simulink model "Rear_SUS_S"  (R2014a)
settings: Solver=ode3  StartTime=0.0  StopTime=T  FixedStep=0.1  RelTol=1e-3
values from neighbouring files (symbols this model uses):
  CA = str2double(get(handles.CA,'string'))    [Rear_SUS.m]    (also in Rear_SUS_GUI.m)
  IN = str2double(get(handles.IN,'string'))    [Rear_SUS.m]    (also in Rear_SUS_GUI.m)
  LT = str2double(get(handles.LT,'string'))    [Rear_SUS_GUI.m]
  N = 1    [Rear_SUS.m]
  Rty = 0    [Rear_SUS_GUI.m]
  Rtz = 0    [Rear_SUS_GUI.m]
  SR = str2double(get(handles.SR,'string'))    [Rear_SUS.m]    (also in Rear_SUS_GUI.m)
  T5 = str2double(get(handles.T5,'string'))    [Rear_SUS.m]    (also in Rear_SUS_GUI.m)
  T6 = str2double(get(handles.T6,'string'))    [Rear_SUS.m]    (also in Rear_SUS_GUI.m)
  X11 = i_x+X6    [Rear_SUS_GUI.m]
  X12 = o_x+X3    [Rear_SUS_GUI.m]
  X14 = X9+X14_1    [Rear_SUS_GUI.m]
  X15 = X9+X15_1    [Rear_SUS_GUI.m]
  X16 = X9+X16_2    [Rear_SUS_GUI.m]
  X2 = L-abs(Z3)*tand(CA)    [Rear_SUS_GUI.m]
  x2 = x4    [Rear_SUS_GUI.m]
  X3 = L+abs(Z2)*tand(CA)    [Rear_SUS_GUI.m]
  x3 = 0    [Rear_SUS_GUI.m]
  x4 = str2double(get(handles.x4,'string'))    [Rear_SUS.m]    (also in Rear_SUS_GUI.m)
  X5 = X4-a1*cosd(T5)    [Rear_SUS_GUI.m]
  x5 = 0    [Rear_SUS_GUI.m]
  X6 = X4+b1*cosd(T5)    [Rear_SUS_GUI.m]
  X7 = X1-a2*cosd(T6)    [Rear_SUS_GUI.m]
  x7 = 0    [Rear_SUS_GUI.m]
  x8 = x8(n)    [Rear_SUS_GUI.m]
  X8 = X1+b2*cosd(T6)    [Rear_SUS_GUI.m]
  x9 = str2double(get(handles.x9,'string'))    [Rear_SUS.m]    (also in Rear_SUS_GUI.m)
  X9 = str2double(get(handles.X9,'string'))    [Rear_SUS.m]    (also in Rear_SUS_GUI.m)
  Y11 = Y6    [Rear_SUS_GUI.m]
  Y12 = Y3    [Rear_SUS_GUI.m]
  Y14 = Y9+Y14_1    [Rear_SUS_GUI.m]
  Y15 = Y9+Y15_1    [Rear_SUS_GUI.m]
  Y16 = Y9+Y16_2    [Rear_SUS_GUI.m]
  Y2 = (Z2-Z9)/K2_3+Y9-SR    [Rear_SUS_GUI.m]
  y2 = Y1+l2*cosd(t2+T2)    [Rear_SUS_GUI.m]
  Y3 = (Z3-Z9)/K2_3+Y9-SR    [Rear_SUS_GUI.m]
  y3 = l4*cosd(t4)    [Rear_SUS_GUI.m]
  y4 = str2double(get(handles.y4,'string'))    [Rear_SUS.m]    (also in Rear_SUS_GUI.m)
  Y5 = Y4    [Rear_SUS_GUI.m]
  y5 = l5*cosd(t5)    [Rear_SUS_GUI.m]
  Y6 = Y4    [Rear_SUS_GUI.m]
  Y7 = Y1    [Rear_SUS_GUI.m]
  y7 = l7*cosd(t7)    [Rear_SUS_GUI.m]
  y8 = y9    [Rear_SUS_GUI.m]
  Y8 = Y1    [Rear_SUS_GUI.m]
  y9 = y7+y4    [Rear_SUS_GUI.m]
  Y9 = str2double(get(handles.Y9,'string'))    [Rear_SUS.m]    (also in Rear_SUS_GUI.m)
  Z11 = Z6    [Rear_SUS_GUI.m]
  Z12 = Z3    [Rear_SUS_GUI.m]
  Z14 = Z9+Z14_1    [Rear_SUS_GUI.m]
  Z15 = Z9+Z15_1    [Rear_SUS_GUI.m]
  Z16 = Z9+Z16_2    [Rear_SUS_GUI.m]
  Z2 = str2double(get(handles.Z2,'string'))    [Rear_SUS.m]    (also in Rear_SUS_GUI.m)
  z2 = Z1+l2*sind(t2+T2)    [Rear_SUS_GUI.m]
  Z3 = str2double(get(handles.Z3,'string'))    [Rear_SUS.m]    (also in Rear_SUS_GUI.m)
  z3 = l4*sind(t4)    [Rear_SUS_GUI.m]
  z4 = str2double(get(handles.z4,'string'))    [Rear_SUS.m]    (also in Rear_SUS_GUI.m)
  Z5 = Z4-a1*sind(T5)    [Rear_SUS_GUI.m]
  z5 = l5*sind(t5)    [Rear_SUS_GUI.m]
  Z6 = Z4+b1*sind(T5)    [Rear_SUS_GUI.m]
  Z7 = Z1-a2*sind(T6)    [Rear_SUS_GUI.m]
  z7 = l7*sind(t7)    [Rear_SUS_GUI.m]
  z8 = z8(n)    [Rear_SUS_GUI.m]
  Z8 = Z1+b2*sind(T6)    [Rear_SUS_GUI.m]
  z9 = str2double(get(handles.z9,'string'))    [Rear_SUS.m]    (also in Rear_SUS_GUI.m)
  Z9 = str2double(get(handles.Z9,'string'))    [Rear_SUS.m]    (also in Rear_SUS_GUI.m)
libraries: mblibv1 x45, simulink x1
settings Model: Creator=ZBingF  LastModifiedBy=ZBingF
settings SimMechanicsCC: VisDuringSimulation=on

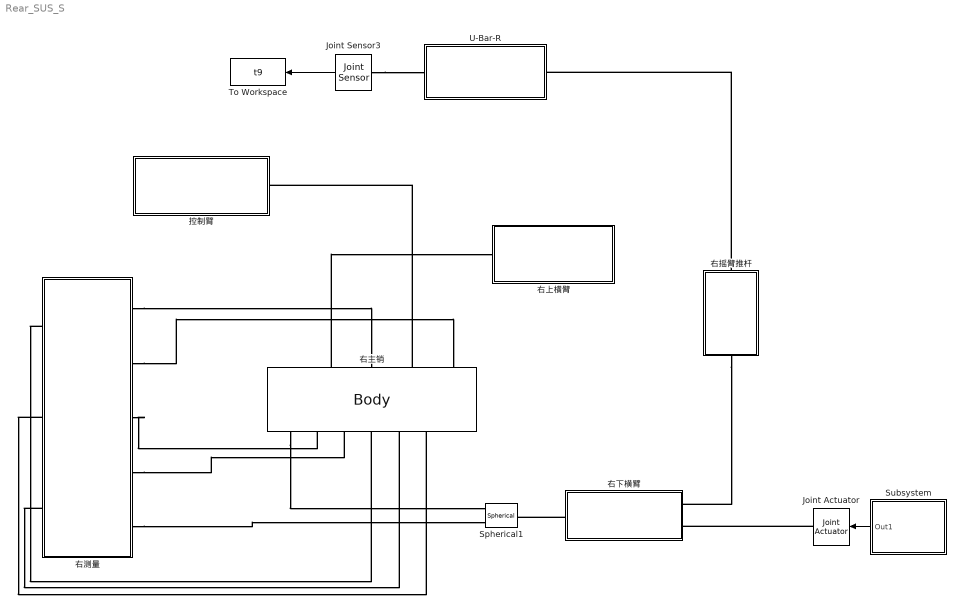
== system Rear_SUS_S ==
  Joint Actuator : mblibv1/Sensors &  Actuators/Joint Actuator  UpdateFromCAD=off  PhysicalDomain=Mechanical  PortType=blob  ActuationStyle=Motion  AngleUnits=deg  ArcVelocityUnits=deg/s  ArcAccelerationUnits=deg/s^2  CoordPositionUnits=m  VelocityUnits=m/s  AccelerationUnits=m/s^2  ForceUnits=N  TorqueUnits=N*m  ActiveIO=on  Width=3  DialogClass=MechanicalActuatorBlock  Primitive=R1  ReferenceFrame=Absolute (World)
  Joint Sensor3 : mblibv1/Sensors &  Actuators/Joint Sensor  RequirementInfo={} %GIDa_0a7a8ca0_e337_4e76_abf1_cf09af27d72f  UpdateFromCAD=off  PhysicalDomain=Mechanical  PortType=blob  Muxed=on  Pose=off  Angle=on  AngleUnits=deg  ArcVelocity=off  ArcVelocityUnits=deg/s  ArcAcceleration=off  ArcAccelerationUnits=deg/s^2  CoordPosition=on  CoordPositionUnits=m  Velocity=off  VelocityUnits=m/s  Acceleration=off  AccelerationUnits=m/s^2  Quaternion=on  QuaternionDT=off  QuaternionDDT=off  QuaternionUnits=off  OutputVector=[1]  ActiveIO=on  Width=1  DialogClass=MechanicalSensorBlock  Primitive=R1  Force=off  ForceUnits=N  Torque=off  TorqueUnits=N*m  ReferenceFrame=Absolute (World)  ReactionSensedSide=Follower  ReactionReferenceFrame=Local (Body CS)  ReactionForce=off  ReactionForceUnits=N  ReactionMoment=off  ReactionMomentUnits=N*m
  Spherical1 : mblibv1/Joints/Spherical  LConnTagsString=__newl0|SA1  RConnTagsString=__newr0  UpdateFromCAD=off  NumSAPorts=1  CutJoint=off  MarkAsCut=off  Primitives=spherical  PrimitiveProps=S$World$[0 0 0]$spherical  DialogClass=JointBlock  SAxis=[0 0 0]
  Subsystem : Subsystem
  To Workspace : ToWorkspace  VariableName=t9  SampleTime=-1
      settings: RequirementInfo={} %GIDa_d72a3179_2628_430b_b3d8_b1966fbe8101
  U-Bar-R : Subsystem
  右上横臂 : Subsystem
  右下横臂 : Subsystem
  右主销 : mblibv1/Bodies/Body  LConnTagsString=CG|CS1|CS4|CS6|CS7  RConnTagsString=CS2|CS5|CS3|CS10|CS12|CS11|CS9  UpdateFromCAD=off  DialogClass=MechanicalBodyBlock  Mass=1  MassUnits=kg  InertiaUnits=kg*m^2  Inertia=eye(3)  Shape=Cylinder  ShapeDims=[1 1]  ShapeUnits=m  ShapeUse=false  Density=1  DensityUnits=kg/m^3  DensityUse=false  GraphicsMode=MACHINE_DEFAULT  BodyColorSelMode=MACHINE_DEFAULT  BodyColor=[1 0 0]  AttachedToCS=CG  CG=Left$CG$[X2 Y2 Z2]$WORLD$WORLD$mm$[0 0 0]$Euler X-Y-Z$deg$WORLD$true$none  WorkingFrames=Left$CS1$[X3 Y3 Z3]$World$World$mm$[0 0 0]$Euler X-Y-Z$deg$WORLD$true$none#Left$CS4$[X3 Y3 Z3]$World$World$mm$[0 0 0]$Euler X-Y-Z$deg$WORLD$true$none#Right$CS2$[X2 Y2 Z2]$World$World$mm$[IN CA 0]$Euler X-Y-Z$deg$WORLD$true$none#Right$CS5$[X2 Y2 Z2]$World$World$mm$[0 0 0]$Euler X-Y-Z$deg$WORLD$true$none#Right$CS3$[X9 Y9 Z9]$World$World$mm$[0 0 0]$Euler X-Y-Z$deg$WORLD$true$none#Right$CS10$[X14 Y14 Z14]$World$World$mm$[0 0 0]$Euler X-Y-Z$deg$WORLD$true$none#Right$CS12$[X16 Y16 Z16]$World$World$mm$[0 0 0]$Euler X-Y-Z$deg$WORLD$true$none#Right$CS11$[X15 Y15 Z15]$World$World$mm$[0 0 0]$Euler X-Y-Z$deg$WORLD$true$none#Right$CS9$[X9 Y9-SR Z9]$World$World$mm$[IN CA 0]$Euler X-Y-Z$deg$WORLD$true$none#Left$CS6$[X12 Y12 Z12]$World$World$mm$[0 0 0]$Euler X-Y-Z$deg$WORLD$true$none#Left$CS7$[X12 Y12 Z12]$World$World$mm$[0 0 0]$Euler X-Y-Z$deg$WORLD$true$none  CGPos=[X2 Y2 Z2]  CGRot=[0 0 0]  CS0Pos=[]  CS0Rot=[]  CS1Pos=[X3 Y3 Z3]  CS1Rot=[0 0 0]  CS2Pos=[X2 Y2 Z2]  CS2Rot=[IN CA 0]  CS3Pos=[X9 Y9 Z9]  CS3Rot=[0 0 0]  CS4Pos=[X3 Y3 Z3]  CS4Rot=[0 0 0]  CS5Pos=[X2 Y2 Z2]  CS5Rot=[0 0 0]  CS6Pos=[X12 Y12 Z12]  CS6Rot=[0 0 0]  CS7Pos=[X12 Y12 Z12]  CS7Rot=[0 0 0]  CS8Pos=[]  CS8Rot=[]  CS9Pos=[X9 Y9-SR Z9]  CS9Rot=[IN CA 0]  CS10Pos=[X14 Y14 Z14]  CS10Rot=[0 0 0]  CS11Pos=[X15 Y15 Z15]  CS11Rot=[0 0 0]  CS12Pos=[X16 Y16 Z16]  CS12Rot=[0 0 0]  CS13Pos=[]  CS13Rot=[]  CS14Pos=[]  CS14Rot=[]  CS15Pos=[]  CS15Rot=[]  CS16Pos=[]  CS16Rot=[]  CS17Pos=[]  CS17Rot=[]  CS18Pos=[]  CS18Rot=[]  CS19Pos=[]  CS19Rot=[]  CS20Pos=[]  CS20Rot=[]
  右摇臂推杆 : Subsystem
  右测量 : Subsystem
  控制臂 : Subsystem
  wires:
  Subsystem/1(Out1) -> Joint Actuator/1
  Joint Sensor3/1 -> To Workspace/1
  connections:
  右主销/RConn1 -- Spherical1/LConn1
  右主销/LConn4 -- 控制臂/RConn1
  右主销/LConn2 -- 右上横臂/LConn1
  右摇臂推杆/RConn1 -- 右下横臂/LConn1
  右下横臂/RConn1 -- Spherical1/RConn1
  Joint Actuator/RConn1 -- 右下横臂/LConn2
  右测量/RConn1 -- 右主销/LConn3
  右测量/RConn2 -- 右主销/LConn5
  右测量/RConn3 -- 右主销/RConn2
  右测量/RConn4 -- 右主销/RConn3
  右测量/RConn5 -- Spherical1/LConn2
  右测量/LConn1 -- 右主销/RConn4
  右测量/LConn2 -- 右主销/RConn6
  右测量/LConn3 -- 右主销/RConn5
  右摇臂推杆/LConn1 -- U-Bar-R/LConn1
  Joint Sensor3/LConn1 -- U-Bar-R/RConn1

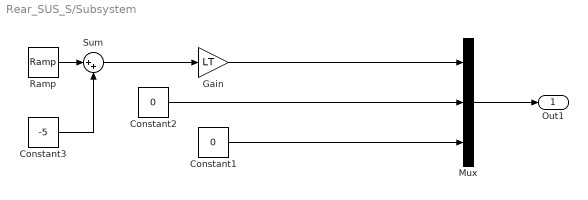
== system Rear_SUS_S/Subsystem ==
  Constant1 : Constant  Value=0
  Constant2 : Constant  Value=0
  Constant3 : Constant  Value=-5
  Gain : Gain  Gain=LT
  Mux : Mux  Inputs=3
  Ramp : simulink/Sources/Ramp  slope=1  start=0  X0=0
  Sum : Sum  Inputs=|++
  Out1 : Outport
  wires:
  Mux/1 -> Out1/1
  Gain/1 -> Mux/1
  Constant1/1 -> Mux/3
  Constant2/1 -> Mux/2
  Ramp/1 -> Sum/1
  Constant3/1 -> Sum/2
  Sum/1 -> Gain/1

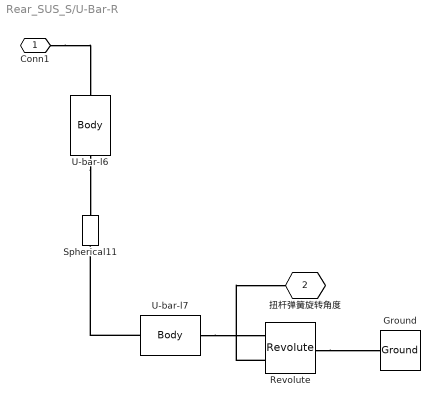
== system Rear_SUS_S/U-Bar-R ==
  Ground : mblibv1/Bodies/Ground  UpdateFromCAD=off  LeftPortType=env  RightPortType=workingframe  PhysicalDomain=Mechanical  DialogClass=GroundBlock  CoordPosition=[x9 y9 z9]  CoordPositionUnits=mm  StateVectorMgrId=-1  MachineId=[0 0]  ShowEnvPort=off  ParameterChecksum=[0 0 0 0]  TopologyChecksum=[0 0 0 0]
  Revolute : mblibv1/Joints/Revolute  LConnTagsString=__newl0|SA1  RConnTagsString=__newr0  UpdateFromCAD=off  NumSAPorts=1  CutJoint=off  MarkAsCut=off  Primitives=prismatic  PrimitiveProps=R1$World$[0 1 0]$revolute  DialogClass=JointBlock  R1Axis=[0 1 0]
  Spherical11 : mblibv1/Joints/Spherical  LConnTagsString=__newl0  RConnTagsString=__newr0  UpdateFromCAD=off  NumSAPorts=0  CutJoint=off  MarkAsCut=off  Primitives=spherical  PrimitiveProps=S$WORLD$[0 0 0]$spherical  DialogClass=JointBlock  SAxis=[0 0 0]
  U-bar-l6 : mblibv1/Bodies/Body  LConnTagsString=CS1  RConnTagsString=CS2  UpdateFromCAD=off  DialogClass=MechanicalBodyBlock  Mass=1  MassUnits=kg  InertiaUnits=kg*m^2  Inertia=eye(3)  Shape=Cylinder  ShapeDims=[1 1]  ShapeUnits=m  ShapeUse=false  Density=1  DensityUnits=kg/m^3  DensityUse=false  GraphicsMode=MACHINE_DEFAULT  BodyColorSelMode=MACHINE_DEFAULT  BodyColor=[1 0 0]  AttachedToCS=CG  CG=Left$CG$[x8 y8 z8]$WORLD$WORLD$mm$[0 0 0]$Euler X-Y-Z$deg$WORLD$false$none  WorkingFrames=Left$CS1$[x8 y8 z8]$World$World$mm$[0 0 0]$Euler X-Y-Z$deg$WORLD$true$none#Right$CS2$[0 0 0]$Adjoining$Adjoining$mm$[0 0 0]$Euler X-Y-Z$deg$WORLD$true$none  CGPos=[x8 y8 z8]  CGRot=[0 0 0]  CS0Pos=[]  CS0Rot=[]  CS1Pos=[x8 y8 z8]  CS1Rot=[0 0 0]  CS2Pos=[0 0 0]  CS2Rot=[0 0 0]  CS3Pos=[]  CS3Rot=[]  CS4Pos=[]  CS4Rot=[]  CS5Pos=[]  CS5Rot=[]  CS6Pos=[]  CS6Rot=[]  CS7Pos=[]  CS7Rot=[]  CS8Pos=[]  CS8Rot=[]  CS9Pos=[]  CS9Rot=[]  CS10Pos=[]  CS10Rot=[]  CS11Pos=[]  CS11Rot=[]  CS12Pos=[]  CS12Rot=[]  CS13Pos=[]  CS13Rot=[]  CS14Pos=[]  CS14Rot=[]  CS15Pos=[]  CS15Rot=[]  CS16Pos=[]  CS16Rot=[]  CS17Pos=[]  CS17Rot=[]  CS18Pos=[]  CS18Rot=[]  CS19Pos=[]  CS19Rot=[]  CS20Pos=[]  CS20Rot=[]
  U-bar-l7 : mblibv1/Bodies/Body  LConnTagsString=CS1  RConnTagsString=CS2  UpdateFromCAD=off  DialogClass=MechanicalBodyBlock  Mass=1  MassUnits=kg  InertiaUnits=kg*m^2  Inertia=eye(3)  Shape=Cylinder  ShapeDims=[1 1]  ShapeUnits=m  ShapeUse=false  Density=1  DensityUnits=kg/m^3  DensityUse=false  GraphicsMode=MACHINE_DEFAULT  BodyColorSelMode=MACHINE_DEFAULT  BodyColor=[1 0 0]  AttachedToCS=CG  CG=Left$CG$[(x8+x9)/2 (y8+y9)/2 (z8+z9)/2]$WORLD$WORLD$mm$[0 0 0]$Euler X-Y-Z$deg$WORLD$false$none  WorkingFrames=Left$CS1$[x9 y9 z9]$World$World$mm$[0 0 0]$Euler X-Y-Z$deg$WORLD$true$none#Right$CS2$[x8 y8 z8]$World$World$mm$[0 0 0]$Euler X-Y-Z$deg$WORLD$true$none  CGPos=[(x8+x9)/2 (y8+y9)/2 (z8+z9)/2]  CGRot=[0 0 0]  CS0Pos=[]  CS0Rot=[]  CS1Pos=[x9 y9 z9]  CS1Rot=[0 0 0]  CS2Pos=[x8 y8 z8]  CS2Rot=[0 0 0]  CS3Pos=[]  CS3Rot=[]  CS4Pos=[]  CS4Rot=[]  CS5Pos=[]  CS5Rot=[]  CS6Pos=[]  CS6Rot=[]  CS7Pos=[]  CS7Rot=[]  CS8Pos=[]  CS8Rot=[]  CS9Pos=[]  CS9Rot=[]  CS10Pos=[]  CS10Rot=[]  CS11Pos=[]  CS11Rot=[]  CS12Pos=[]  CS12Rot=[]  CS13Pos=[]  CS13Rot=[]  CS14Pos=[]  CS14Rot=[]  CS15Pos=[]  CS15Rot=[]  CS16Pos=[]  CS16Rot=[]  CS17Pos=[]  CS17Rot=[]  CS18Pos=[]  CS18Rot=[]  CS19Pos=[]  CS19Rot=[]  CS20Pos=[]  CS20Rot=[]
  Conn1 : PMIOPort  Port=1  Side=Left
  扭杆弹簧旋转角度 : PMIOPort  Port=2  Side=Right
  connections:
  U-bar-l6/LConn1 -- Spherical11/RConn1
  U-bar-l7/RConn1 -- Spherical11/LConn1
  Conn1/RConn1 -- U-bar-l6/RConn1
  U-bar-l7/LConn1 -- Revolute/LConn1
  Revolute/RConn1 -- Ground/RConn1
  Revolute/LConn2 -- 扭杆弹簧旋转角度/RConn1

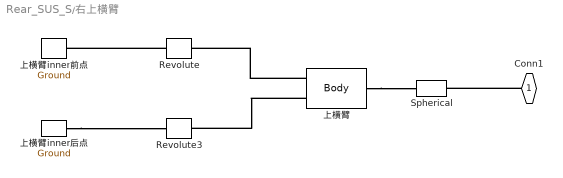
== system Rear_SUS_S/右上横臂 ==
  Revolute : mblibv1/Joints/Revolute  LConnTagsString=__newl0  RConnTagsString=__newr0  UpdateFromCAD=off  NumSAPorts=0  CutJoint=off  MarkAsCut=off  Primitives=prismatic  PrimitiveProps=R1$World$[cosd(T5) 0 sind(T5)]$revolute  DialogClass=JointBlock  R1Axis=[cosd(T5) 0 sind(T5)]
  Revolute3 : mblibv1/Joints/Revolute  LConnTagsString=__newl0  RConnTagsString=__newr0  UpdateFromCAD=off  NumSAPorts=0  CutJoint=off  MarkAsCut=off  Primitives=prismatic  PrimitiveProps=R1$World$[cosd(T5) 0 sind(T5)]$revolute  DialogClass=JointBlock  R1Axis=[cosd(T5) 0 sind(T5)]
  Spherical : mblibv1/Joints/Spherical  LConnTagsString=__newl0  RConnTagsString=__newr0  UpdateFromCAD=off  NumSAPorts=0  CutJoint=off  MarkAsCut=off  Primitives=spherical  PrimitiveProps=S$World$[0 0 0]$spherical  DialogClass=JointBlock  SAxis=[0 0 0]
  上横臂 : mblibv1/Bodies/Body  LConnTagsString=CS1|CS3  RConnTagsString=CS2  UpdateFromCAD=off  DialogClass=MechanicalBodyBlock  Mass=1  MassUnits=kg  InertiaUnits=kg*m^2  Inertia=eye(3)  Shape=Cylinder  ShapeDims=[1 1]  ShapeUnits=m  ShapeUse=false  Density=1  DensityUnits=kg/m^3  DensityUse=false  GraphicsMode=MACHINE_DEFAULT  BodyColorSelMode=MACHINE_DEFAULT  BodyColor=[1 0 0]  AttachedToCS=CG  CG=Left$CG$[X3 Y3 Z3]$WORLD$WORLD$mm$[0 0 0]$Euler X-Y-Z$deg$WORLD$false$none  WorkingFrames=Left$CS1$[X5 Y5 Z5]$World$World$mm$[0 0 0]$Euler X-Y-Z$deg$WORLD$true$none#Right$CS2$[X3 Y3 Z3]$World$World$mm$[0 0 0]$Euler X-Y-Z$deg$WORLD$true$none#Left$CS3$[X6 Y6 Z6]$World$World$mm$[0 0 0]$Euler X-Y-Z$deg$WORLD$true$none  CGPos=[X3 Y3 Z3]  CGRot=[0 0 0]  CS0Pos=[]  CS0Rot=[]  CS1Pos=[X5 Y5 Z5]  CS1Rot=[0 0 0]  CS2Pos=[X3 Y3 Z3]  CS2Rot=[0 0 0]  CS3Pos=[X6 Y6 Z6]  CS3Rot=[0 0 0]  CS4Pos=[]  CS4Rot=[]  CS5Pos=[]  CS5Rot=[]  CS6Pos=[]  CS6Rot=[]  CS7Pos=[]  CS7Rot=[]  CS8Pos=[]  CS8Rot=[]  CS9Pos=[]  CS9Rot=[]  CS10Pos=[]  CS10Rot=[]  CS11Pos=[]  CS11Rot=[]  CS12Pos=[]  CS12Rot=[]  CS13Pos=[]  CS13Rot=[]  CS14Pos=[]  CS14Rot=[]  CS15Pos=[]  CS15Rot=[]  CS16Pos=[]  CS16Rot=[]  CS17Pos=[]  CS17Rot=[]  CS18Pos=[]  CS18Rot=[]  CS19Pos=[]  CS19Rot=[]  CS20Pos=[]  CS20Rot=[]
  上横臂inner前点 : mblibv1/Bodies/Ground  UpdateFromCAD=off  LeftPortType=env  RightPortType=workingframe  PhysicalDomain=Mechanical  DialogClass=GroundBlock  CoordPosition=[X5 Y5 Z5]  CoordPositionUnits=mm  StateVectorMgrId=-1  MachineId=[0 0]  ShowEnvPort=off  ParameterChecksum=[0 0 0 0]  TopologyChecksum=[0 0 0 0]
  上横臂inner后点 : mblibv1/Bodies/Ground  UpdateFromCAD=off  LeftPortType=env  RightPortType=workingframe  PhysicalDomain=Mechanical  DialogClass=GroundBlock  CoordPosition=[X6 Y6 Z6]  CoordPositionUnits=mm  StateVectorMgrId=-1  MachineId=[0 0]  ShowEnvPort=off  ParameterChecksum=[0 0 0 0]  TopologyChecksum=[0 0 0 0]
  Conn1 : PMIOPort  Port=1  Side=Left
  connections:
  Revolute/LConn1 -- 上横臂inner前点/RConn1
  上横臂/RConn1 -- Spherical/LConn1
  Conn1/RConn1 -- Spherical/RConn1
  上横臂/LConn2 -- Revolute3/RConn1
  上横臂inner后点/RConn1 -- Revolute3/LConn1
  上横臂/LConn1 -- Revolute/RConn1

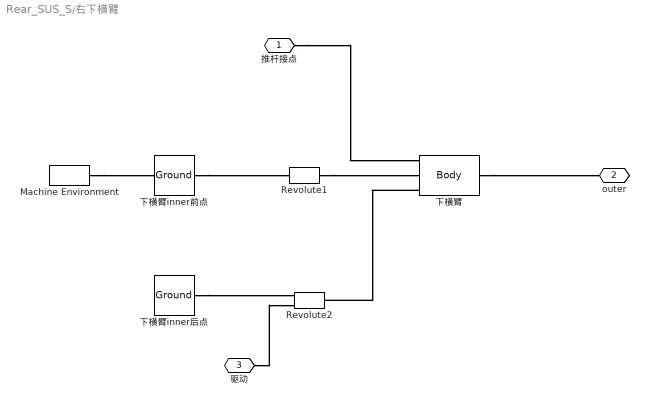
== system Rear_SUS_S/右下横臂 ==
  Machine Environment : mblibv1/Bodies/Machine Environment  PortType=env  PhysicalDomain=Mechanical  DialogTemplateClass=MECH.MachineEnvironment  SyncWhenCopied=off  Gravity=[0 0 -9.81]  GravityUnits=m/s^2  GravityAsSignal=off  Dimensionality=Auto-detect  AnalysisType=Forward dynamics  LinearAssemblyTolerance=1e-3  LinearAssemblyToleranceUnits=m  AngularAssemblyTolerance=1e-3  AngularAssemblyToleranceUnits=rad  ConstraintSolverType=Stabilizing  ConstraintRelTolerance=1e-4  ConstraintAbsTolerance=1e-4  UseRobustSingularityHandling=off  RedundancyAnalysisToleranceType=Automatically select tolerance  RedundancyAnalysisTolerance=1e-14  StatePerturbationType=Fixed  PerturbationSize=1e-5  VisualizeMachine=on  BodyVisualizationType=Use model default body geometries  BodyColorSelMode=Use model default  DefaultBodyColor=[1 0 0]
  Revolute1 : mblibv1/Joints/Revolute  LConnTagsString=__newl0  RConnTagsString=__newr0  UpdateFromCAD=off  NumSAPorts=0  CutJoint=off  MarkAsCut=off  Primitives=prismatic  PrimitiveProps=R1$World$[cosd(T6) 0 sind(T6)]$revolute  DialogClass=JointBlock  R1Axis=[cosd(T6) 0 sind(T6)]
  Revolute2 : mblibv1/Joints/Revolute  LConnTagsString=__newl0|SA1  RConnTagsString=__newr0  UpdateFromCAD=off  NumSAPorts=1  CutJoint=off  MarkAsCut=off  Primitives=prismatic  PrimitiveProps=R1$World$[cosd(T6) 0 sind(T6)]$revolute  DialogClass=JointBlock  R1Axis=[cosd(T6) 0 sind(T6)]
  下横臂 : mblibv1/Bodies/Body  LConnTagsString=CS3|CS1|CS4  RConnTagsString=CS2  UpdateFromCAD=off  DialogClass=MechanicalBodyBlock  Mass=1  MassUnits=kg  InertiaUnits=kg*m^2  Inertia=eye(3)  Shape=Cylinder  ShapeDims=[1 1]  ShapeUnits=m  ShapeUse=false  Density=1  DensityUnits=kg/m^3  DensityUse=false  GraphicsMode=MACHINE_DEFAULT  BodyColorSelMode=MACHINE_DEFAULT  BodyColor=[1 0 0]  AttachedToCS=CG  CG=Left$CG$[X2 Y2 Z2]$WORLD$WORLD$mm$[0 0 0]$Euler X-Y-Z$deg$WORLD$false$none  WorkingFrames=Left$CS3$[x2 y2 z2]$WORLD$WORLD$mm$[0 0 0]$Euler X-Y-Z$deg$WORLD$true$none#Left$CS1$[X7 Y7 Z7]$World$World$mm$[0 0 0]$Euler X-Y-Z$deg$WORLD$true$none#Right$CS2$[X2 Y2 Z2]$World$World$mm$[IN CA 0]$Euler X-Y-Z$deg$WORLD$true$none#Left$CS4$[X8 Y8 Z8]$World$World$mm$[0 0 0]$Euler X-Y-Z$deg$WORLD$true$none  CGPos=[X2 Y2 Z2]  CGRot=[0 0 0]  CS0Pos=[]  CS0Rot=[]  CS1Pos=[X7 Y7 Z7]  CS1Rot=[0 0 0]  CS2Pos=[X2 Y2 Z2]  CS2Rot=[IN CA 0]  CS3Pos=[x2 y2 z2]  CS3Rot=[0 0 0]  CS4Pos=[X8 Y8 Z8]  CS4Rot=[0 0 0]  CS5Pos=[]  CS5Rot=[]  CS6Pos=[]  CS6Rot=[]  CS7Pos=[]  CS7Rot=[]  CS8Pos=[]  CS8Rot=[]  CS9Pos=[]  CS9Rot=[]  CS10Pos=[]  CS10Rot=[]  CS11Pos=[]  CS11Rot=[]  CS12Pos=[]  CS12Rot=[]  CS13Pos=[]  CS13Rot=[]  CS14Pos=[]  CS14Rot=[]  CS15Pos=[]  CS15Rot=[]  CS16Pos=[]  CS16Rot=[]  CS17Pos=[]  CS17Rot=[]  CS18Pos=[]  CS18Rot=[]  CS19Pos=[]  CS19Rot=[]  CS20Pos=[]  CS20Rot=[]
  下横臂inner前点 : mblibv1/Bodies/Ground  UpdateFromCAD=off  LeftPortType=env  RightPortType=workingframe  PhysicalDomain=Mechanical  DialogClass=GroundBlock  CoordPosition=[X7 Y7 Z7]  CoordPositionUnits=mm  StateVectorMgrId=0  MachineId=[1 0]  ShowEnvPort=on  ParameterChecksum=[1663249025, 2754832369, 2702422240, 986948338]  TopologyChecksum=[3704747193, 758239368, 2115105119, 2031816838]
  下横臂inner后点 : mblibv1/Bodies/Ground  UpdateFromCAD=off  LeftPortType=env  RightPortType=workingframe  PhysicalDomain=Mechanical  DialogClass=GroundBlock  CoordPosition=[X8 Y8 Z8]  CoordPositionUnits=mm  StateVectorMgrId=-1  MachineId=[0 0]  ShowEnvPort=off  ParameterChecksum=[0 0 0 0]  TopologyChecksum=[0 0 0 0]
  推杆接点 : PMIOPort  Port=1  Side=Left
  outer : PMIOPort  Port=2  Side=Right
  驱动 : PMIOPort  Port=3  Side=Left
  connections:
  下横臂/RConn1 -- outer/RConn1
  Revolute1/RConn1 -- 下横臂/LConn2
  下横臂inner后点/RConn1 -- Revolute2/LConn1
  Machine Environment/RConn1 -- 下横臂inner前点/LConn1
  下横臂/LConn3 -- Revolute2/RConn1
  下横臂inner前点/RConn1 -- Revolute1/LConn1
  驱动/RConn1 -- Revolute2/LConn2
  推杆接点/RConn1 -- 下横臂/LConn1

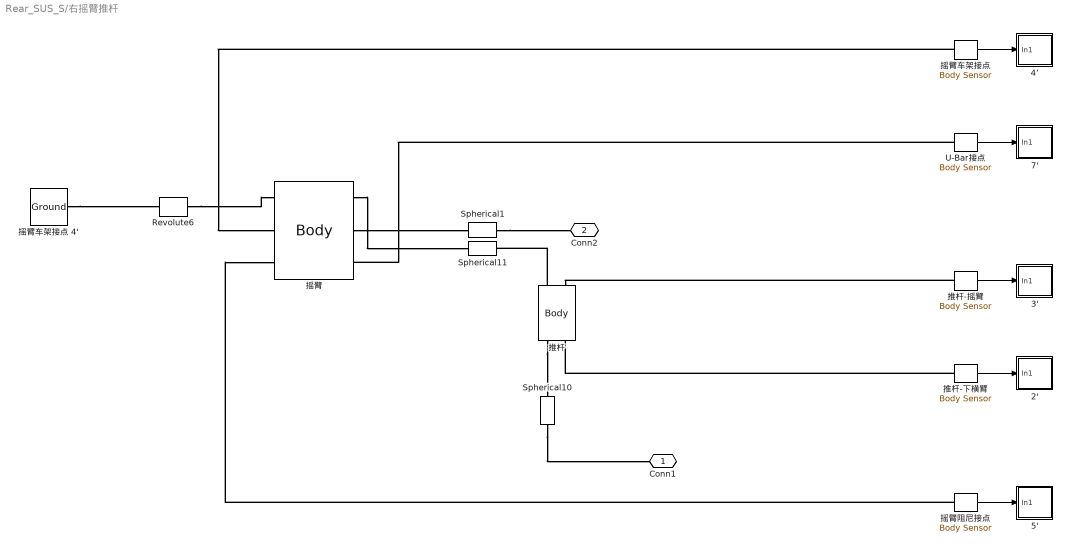
== system Rear_SUS_S/右摇臂推杆 ==
  2' : Subsystem
  3' : Subsystem
  4’ : Subsystem
  5' : Subsystem
  7' : Subsystem
  Revolute6 : mblibv1/Joints/Revolute  LConnTagsString=__newl0  RConnTagsString=__newr0  UpdateFromCAD=off  NumSAPorts=0  CutJoint=off  MarkAsCut=off  Primitives=prismatic  PrimitiveProps=R1$Follower$[1 0 0]$revolute  DialogClass=JointBlock  R1Axis=[1 0 0]
  Spherical1 : mblibv1/Joints/Spherical  LConnTagsString=__newl0  RConnTagsString=__newr0  UpdateFromCAD=off  NumSAPorts=0  CutJoint=off  MarkAsCut=off  Primitives=spherical  PrimitiveProps=S$World$[0 0 0]$spherical  DialogClass=JointBlock  SAxis=[0 0 0]
  Spherical10 : mblibv1/Joints/Spherical  LConnTagsString=__newl0  RConnTagsString=__newr0  UpdateFromCAD=off  NumSAPorts=0  CutJoint=off  MarkAsCut=off  Primitives=spherical  PrimitiveProps=S$WORLD$[0 0 0]$spherical  DialogClass=JointBlock  SAxis=[0 0 0]
  Spherical11 : mblibv1/Joints/Spherical  LConnTagsString=__newl0  RConnTagsString=__newr0  UpdateFromCAD=off  NumSAPorts=0  CutJoint=off  MarkAsCut=off  Primitives=spherical  PrimitiveProps=S$WORLD$[0 0 0]$spherical  DialogClass=JointBlock  SAxis=[0 0 0]
  U-Bar接点 : mblibv1/Sensors &  Actuators/Body Sensor  UpdateFromCAD=off  PhysicalDomain=Mechanical  PortType=blob  Muxed=on  Pose=off  Angle=on  AngleUnits=deg  ArcVelocity=off  ArcVelocityUnits=deg/s  ArcAcceleration=off  ArcAccelerationUnits=deg/s^2  CoordPosition=on  CoordPositionUnits=mm  Velocity=off  VelocityUnits=mm/s  Acceleration=off  AccelerationUnits=m/s^2  Quaternion=on  QuaternionDT=off  QuaternionDDT=off  QuaternionUnits=off  OutputVector=[1]  ActiveIO=off  Width=3  DialogClass=MechanicalSensorBlock  ReferenceFrame=Absolute (World)
  推杆 : mblibv1/Bodies/Body  LConnTagsString=CS1|CS4  RConnTagsString=CS2|CS3  UpdateFromCAD=off  DialogClass=MechanicalBodyBlock  Mass=1  MassUnits=kg  InertiaUnits=kg*m^2  Inertia=eye(3)  Shape=Cylinder  ShapeDims=[1 1]  ShapeUnits=m  ShapeUse=false  Density=1  DensityUnits=kg/m^3  DensityUse=false  GraphicsMode=MACHINE_DEFAULT  BodyColorSelMode=MACHINE_DEFAULT  BodyColor=[1 0 0]  AttachedToCS=CG  CG=Left$CG$[x2 y2 z2]$WORLD$WORLD$mm$[0 0 0]$Euler X-Y-Z$deg$WORLD$false$none  WorkingFrames=Left$CS1$[x2 y2 z2]$World$World$mm$[0 0 0]$Euler X-Y-Z$deg$WORLD$true$none#Left$CS4$[x2 y2 z2]$World$World$mm$[0 0 0]$Euler X-Y-Z$deg$WORLD$true$none#Right$CS2$[0 0 0]$Adjoining$Adjoining$mm$[0 0 0]$Euler X-Y-Z$deg$WORLD$true$none#Right$CS3$[0 0 0]$Adjoining$Adjoining$mm$[0 0 0]$Euler X-Y-Z$deg$WORLD$true$none  CGPos=[x2 y2 z2]  CGRot=[0 0 0]  CS0Pos=[]  CS0Rot=[]  CS1Pos=[x2 y2 z2]  CS1Rot=[0 0 0]  CS2Pos=[0 0 0]  CS2Rot=[0 0 0]  CS3Pos=[0 0 0]  CS3Rot=[0 0 0]  CS4Pos=[x2 y2 z2]  CS4Rot=[0 0 0]  CS5Pos=[]  CS5Rot=[]  CS6Pos=[]  CS6Rot=[]  CS7Pos=[]  CS7Rot=[]  CS8Pos=[]  CS8Rot=[]  CS9Pos=[]  CS9Rot=[]  CS10Pos=[]  CS10Rot=[]  CS11Pos=[]  CS11Rot=[]  CS12Pos=[]  CS12Rot=[]  CS13Pos=[]  CS13Rot=[]  CS14Pos=[]  CS14Rot=[]  CS15Pos=[]  CS15Rot=[]  CS16Pos=[]  CS16Rot=[]  CS17Pos=[]  CS17Rot=[]  CS18Pos=[]  CS18Rot=[]  CS19Pos=[]  CS19Rot=[]  CS20Pos=[]  CS20Rot=[]
  推杆-下横臂 : mblibv1/Sensors &  Actuators/Body Sensor  UpdateFromCAD=off  PhysicalDomain=Mechanical  PortType=blob  Muxed=on  Pose=off  Angle=on  AngleUnits=deg  ArcVelocity=off  ArcVelocityUnits=deg/s  ArcAcceleration=off  ArcAccelerationUnits=deg/s^2  CoordPosition=on  CoordPositionUnits=mm  Velocity=off  VelocityUnits=mm/s  Acceleration=off  AccelerationUnits=m/s^2  Quaternion=on  QuaternionDT=off  QuaternionDDT=off  QuaternionUnits=off  OutputVector=[1]  ActiveIO=off  Width=3  DialogClass=MechanicalSensorBlock  ReferenceFrame=Absolute (World)
  推杆-摇臂 : mblibv1/Sensors &  Actuators/Body Sensor  UpdateFromCAD=off  PhysicalDomain=Mechanical  PortType=blob  Muxed=on  Pose=off  Angle=on  AngleUnits=deg  ArcVelocity=off  ArcVelocityUnits=deg/s  ArcAcceleration=off  ArcAccelerationUnits=deg/s^2  CoordPosition=on  CoordPositionUnits=mm  Velocity=off  VelocityUnits=mm/s  Acceleration=off  AccelerationUnits=m/s^2  Quaternion=on  QuaternionDT=off  QuaternionDDT=off  QuaternionUnits=off  OutputVector=[1]  ActiveIO=off  Width=3  DialogClass=MechanicalSensorBlock  ReferenceFrame=Absolute (World)
  摇臂 : mblibv1/Bodies/Body  LConnTagsString=CS1|CS6|CS4  RConnTagsString=CS2|CS5|CS3  UpdateFromCAD=off  DialogClass=MechanicalBodyBlock  Mass=1  MassUnits=kg  InertiaUnits=kg*m^2  Inertia=eye(3)  Shape=Cylinder  ShapeDims=[1 1]  ShapeUnits=m  ShapeUse=false  Density=1  DensityUnits=kg/m^3  DensityUse=false  GraphicsMode=MACHINE_DEFAULT  BodyColorSelMode=MACHINE_DEFAULT  BodyColor=[1 0 0]  AttachedToCS=CG  CG=Left$CG$[x4 y4 z4]$WORLD$WORLD$mm$[0 0 0]$Euler X-Y-Z$deg$WORLD$false$none  WorkingFrames=Left$CS1$[x4 y4 z4]$World$World$mm$[Rtz Rty 0]$Euler Z-Y-X$deg$WORLD$true$none#Left$CS6$[x4 y4 z4]$World$World$mm$[Rtz Rty 0]$Euler Z-Y-X$deg$WORLD$true$none#Right$CS2$[x3 y3 z3]$CS1$CS1$mm$[0 0 0]$Euler X-Y-Z$deg$CS1$true$none#Left$CS4$[x5 y5 z5]$CS1$CS1$mm$[0 0 0]$Euler X-Y-Z$deg$CS1$true$none#Right$CS5$[x7 y7 z7]$CS1$CS1$mm$[0 0 0]$Euler X-Y-Z$deg$CS1$true$none#Right$CS3$[x7 y7 z7]$CS1$CS1$mm$[0 0 0]$Euler X-Y-Z$deg$CS1$true$none  CGPos=[x4 y4 z4]  CGRot=[0 0 0]  CS0Pos=[]  CS0Rot=[]  CS1Pos=[x4 y4 z4]  CS1Rot=[Rtz Rty 0]  CS2Pos=[x3 y3 z3]  CS2Rot=[0 0 0]  CS3Pos=[x7 y7 z7]  CS3Rot=[0 0 0]  CS4Pos=[x5 y5 z5]  CS4Rot=[0 0 0]  CS5Pos=[x7 y7 z7]  CS5Rot=[0 0 0]  CS6Pos=[x4 y4 z4]  CS6Rot=[Rtz Rty 0]  CS7Pos=[]  CS7Rot=[]  CS8Pos=[]  CS8Rot=[]  CS9Pos=[]  CS9Rot=[]  CS10Pos=[]  CS10Rot=[]  CS11Pos=[]  CS11Rot=[]  CS12Pos=[]  CS12Rot=[]  CS13Pos=[]  CS13Rot=[]  CS14Pos=[]  CS14Rot=[]  CS15Pos=[]  CS15Rot=[]  CS16Pos=[]  CS16Rot=[]  CS17Pos=[]  CS17Rot=[]  CS18Pos=[]  CS18Rot=[]  CS19Pos=[]  CS19Rot=[]  CS20Pos=[]  CS20Rot=[]
  摇臂车架接点 : mblibv1/Sensors &  Actuators/Body Sensor  UpdateFromCAD=off  PhysicalDomain=Mechanical  PortType=blob  Muxed=on  Pose=off  Angle=on  AngleUnits=deg  ArcVelocity=off  ArcVelocityUnits=deg/s  ArcAcceleration=off  ArcAccelerationUnits=deg/s^2  CoordPosition=on  CoordPositionUnits=mm  Velocity=off  VelocityUnits=mm/s  Acceleration=off  AccelerationUnits=m/s^2  Quaternion=on  QuaternionDT=off  QuaternionDDT=off  QuaternionUnits=off  OutputVector=[1]  ActiveIO=off  Width=3  DialogClass=MechanicalSensorBlock  ReferenceFrame=Absolute (World)
  摇臂车架接点 4' : mblibv1/Bodies/Ground  UpdateFromCAD=off  LeftPortType=env  RightPortType=workingframe  PhysicalDomain=Mechanical  DialogClass=GroundBlock  CoordPosition=[x4 y4 z4]  CoordPositionUnits=mm  StateVectorMgrId=-1  MachineId=[0 0]  ShowEnvPort=off  ParameterChecksum=[0 0 0 0]  TopologyChecksum=[0 0 0 0]
  摇臂阻尼接点 : mblibv1/Sensors &  Actuators/Body Sensor  UpdateFromCAD=off  PhysicalDomain=Mechanical  PortType=blob  Muxed=on  Pose=off  Angle=on  AngleUnits=deg  ArcVelocity=off  ArcVelocityUnits=deg/s  ArcAcceleration=off  ArcAccelerationUnits=deg/s^2  CoordPosition=on  CoordPositionUnits=mm  Velocity=off  VelocityUnits=mm/s  Acceleration=off  AccelerationUnits=m/s^2  Quaternion=on  QuaternionDT=off  QuaternionDDT=off  QuaternionUnits=off  OutputVector=[1]  ActiveIO=on  Width=3  DialogClass=MechanicalSensorBlock  ReferenceFrame=Absolute (World)
  Conn1 : PMIOPort  Port=1  Side=Right
  Conn2 : PMIOPort  Port=2  Side=Left
  wires:
  摇臂阻尼接点/1 -> 5'/1(In1)
  U-Bar接点/1 -> 7'/1(In1)
  推杆-摇臂/1 -> 3'/1(In1)
  摇臂车架接点/1 -> 4’/1(In1)
  推杆-下横臂/1 -> 2'/1(In1)
  connections:
  推杆/RConn1 -- Spherical11/LConn1
  Spherical10/RConn1 -- Conn1/RConn1
  摇臂车架接点 4'/RConn1 -- Revolute6/LConn1
  推杆/LConn1 -- Spherical10/LConn1
  摇臂/RConn1 -- Spherical11/RConn1
  Revolute6/RConn1 -- 摇臂/LConn1
  摇臂阻尼接点/LConn1 -- 摇臂/LConn3
  摇臂/RConn2 -- Spherical1/RConn1
  Spherical1/LConn1 -- Conn2/RConn1
  U-Bar接点/LConn1 -- 摇臂/RConn3
  推杆-摇臂/LConn1 -- 推杆/RConn2
  摇臂车架接点/LConn1 -- 摇臂/LConn2
  推杆-下横臂/LConn1 -- 推杆/LConn2

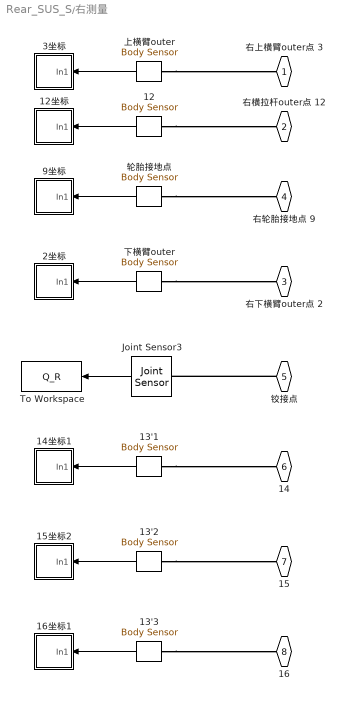
== system Rear_SUS_S/右测量 ==
  " 12" : mblibv1/Sensors &  Actuators/Body Sensor  UpdateFromCAD=off  PhysicalDomain=Mechanical  PortType=blob  Muxed=on  Pose=off  Angle=on  AngleUnits=deg  ArcVelocity=off  ArcVelocityUnits=deg/s  ArcAcceleration=off  ArcAccelerationUnits=deg/s^2  CoordPosition=on  CoordPositionUnits=mm  Velocity=off  VelocityUnits=mm/s  Acceleration=off  AccelerationUnits=m/s^2  Quaternion=on  QuaternionDT=off  QuaternionDDT=off  QuaternionUnits=off  OutputVector=[1]  ActiveIO=on  Width=3  DialogClass=MechanicalSensorBlock  ReferenceFrame=Absolute (World)
  12坐标 : Subsystem
  13'1 : mblibv1/Sensors &  Actuators/Body Sensor  UpdateFromCAD=off  PhysicalDomain=Mechanical  PortType=blob  Muxed=on  Pose=off  Angle=on  AngleUnits=deg  ArcVelocity=off  ArcVelocityUnits=deg/s  ArcAcceleration=off  ArcAccelerationUnits=deg/s^2  CoordPosition=on  CoordPositionUnits=mm  Velocity=off  VelocityUnits=mm/s  Acceleration=off  AccelerationUnits=m/s^2  Quaternion=on  QuaternionDT=off  QuaternionDDT=off  QuaternionUnits=off  OutputVector=[1]  ActiveIO=on  Width=3  DialogClass=MechanicalSensorBlock  ReferenceFrame=Absolute (World)
  13'2 : mblibv1/Sensors &  Actuators/Body Sensor  UpdateFromCAD=off  PhysicalDomain=Mechanical  PortType=blob  Muxed=on  Pose=off  Angle=on  AngleUnits=deg  ArcVelocity=off  ArcVelocityUnits=deg/s  ArcAcceleration=off  ArcAccelerationUnits=deg/s^2  CoordPosition=on  CoordPositionUnits=mm  Velocity=off  VelocityUnits=mm/s  Acceleration=off  AccelerationUnits=m/s^2  Quaternion=on  QuaternionDT=off  QuaternionDDT=off  QuaternionUnits=off  OutputVector=[1]  ActiveIO=on  Width=3  DialogClass=MechanicalSensorBlock  ReferenceFrame=Absolute (World)
  13'3 : mblibv1/Sensors &  Actuators/Body Sensor  UpdateFromCAD=off  PhysicalDomain=Mechanical  PortType=blob  Muxed=on  Pose=off  Angle=on  AngleUnits=deg  ArcVelocity=off  ArcVelocityUnits=deg/s  ArcAcceleration=off  ArcAccelerationUnits=deg/s^2  CoordPosition=on  CoordPositionUnits=mm  Velocity=off  VelocityUnits=mm/s  Acceleration=off  AccelerationUnits=m/s^2  Quaternion=on  QuaternionDT=off  QuaternionDDT=off  QuaternionUnits=off  OutputVector=[1]  ActiveIO=on  Width=3  DialogClass=MechanicalSensorBlock  ReferenceFrame=Absolute (World)
  14坐标1 : Subsystem
  15坐标2 : Subsystem
  16坐标1 : Subsystem
  2坐标 : Subsystem
  3坐标 : Subsystem
  9坐标 : Subsystem
  Joint Sensor3 : mblibv1/Sensors &  Actuators/Joint Sensor  RequirementInfo={} %GIDa_19744d15_74ca_4aeb_a8db_aa456b7a6e07  UpdateFromCAD=off  PhysicalDomain=Mechanical  PortType=blob  Muxed=on  Pose=off  Angle=on  AngleUnits=deg  ArcVelocity=off  ArcVelocityUnits=deg/s  ArcAcceleration=off  ArcAccelerationUnits=deg/s^2  CoordPosition=on  CoordPositionUnits=m  Velocity=off  VelocityUnits=m/s  Acceleration=off  AccelerationUnits=m/s^2  Quaternion=on  QuaternionDT=off  QuaternionDDT=off  QuaternionUnits=off  OutputVector=[1]  ActiveIO=on  Width=4  DialogClass=MechanicalSensorBlock  Primitive=S  Force=off  ForceUnits=N  Torque=off  TorqueUnits=N*m  ReferenceFrame=Absolute (World)  ReactionSensedSide=Follower  ReactionReferenceFrame=Local (Body CS)  ReactionForce=off  ReactionForceUnits=N  ReactionMoment=off  ReactionMomentUnits=N*m
  To Workspace : ToWorkspace  VariableName=Q_R  SampleTime=-1
      settings: RequirementInfo={} %GIDa_08495e0d_609d_4b7e_b26a_a03e3158b1fb
  上横臂outer : mblibv1/Sensors &  Actuators/Body Sensor  UpdateFromCAD=off  PhysicalDomain=Mechanical  PortType=blob  Muxed=on  Pose=off  Angle=on  AngleUnits=deg  ArcVelocity=off  ArcVelocityUnits=deg/s  ArcAcceleration=off  ArcAccelerationUnits=deg/s^2  CoordPosition=on  CoordPositionUnits=mm  Velocity=off  VelocityUnits=mm/s  Acceleration=off  AccelerationUnits=m/s^2  Quaternion=on  QuaternionDT=off  QuaternionDDT=off  QuaternionUnits=off  OutputVector=[1]  ActiveIO=on  Width=3  DialogClass=MechanicalSensorBlock  ReferenceFrame=Absolute (World)
  下横臂outer : mblibv1/Sensors &  Actuators/Body Sensor  UpdateFromCAD=off  PhysicalDomain=Mechanical  PortType=blob  Muxed=on  Pose=off  Angle=on  AngleUnits=deg  ArcVelocity=off  ArcVelocityUnits=deg/s  ArcAcceleration=off  ArcAccelerationUnits=deg/s^2  CoordPosition=on  CoordPositionUnits=mm  Velocity=off  VelocityUnits=mm/s  Acceleration=off  AccelerationUnits=m/s^2  Quaternion=on  QuaternionDT=off  QuaternionDDT=off  QuaternionUnits=off  OutputVector=[1]  ActiveIO=on  Width=3  DialogClass=MechanicalSensorBlock  ReferenceFrame=Absolute (World)
  "轮胎接地点 " : mblibv1/Sensors &  Actuators/Body Sensor  UpdateFromCAD=off  PhysicalDomain=Mechanical  PortType=blob  Muxed=on  Pose=off  Angle=on  AngleUnits=deg  ArcVelocity=off  ArcVelocityUnits=deg/s  ArcAcceleration=off  ArcAccelerationUnits=deg/s^2  CoordPosition=on  CoordPositionUnits=mm  Velocity=off  VelocityUnits=mm/s  Acceleration=off  AccelerationUnits=m/s^2  Quaternion=on  QuaternionDT=off  QuaternionDDT=off  QuaternionUnits=off  OutputVector=[1]  ActiveIO=on  Width=3  DialogClass=MechanicalSensorBlock  ReferenceFrame=Absolute (World)
  右上横臂outer点 3 : PMIOPort  Port=1  Side=Right
  右横拉杆outer点 12 : PMIOPort  Port=2  Side=Right
  右下横臂outer点 2 : PMIOPort  Port=3  Side=Right
  右轮胎接地点 9 : PMIOPort  Port=4  Side=Right
  铰接点 : PMIOPort  Port=5  Side=Right
  14 : PMIOPort  Port=6  Side=Left
  15 : PMIOPort  Port=7  Side=Left
  16 : PMIOPort  Port=8  Side=Left
  wires:
  "轮胎接地点 "/1 -> 9坐标/1(In1)
  上横臂outer/1 -> 3坐标/1(In1)
  下横臂outer/1 -> 2坐标/1(In1)
  " 12"/1 -> 12坐标/1(In1)
  Joint Sensor3/1 -> To Workspace/1
  13'1/1 -> 14坐标1/1(In1)
  13'2/1 -> 15坐标2/1(In1)
  13'3/1 -> 16坐标1/1(In1)
  connections:
  "轮胎接地点 "/LConn1 -- 右轮胎接地点 9/RConn1
  上横臂outer/LConn1 -- 右上横臂outer点 3/RConn1
  下横臂outer/LConn1 -- 右下横臂outer点 2/RConn1
  " 12"/LConn1 -- 右横拉杆outer点 12/RConn1
  铰接点/RConn1 -- Joint Sensor3/LConn1
  13'1/LConn1 -- 14/RConn1
  13'2/LConn1 -- 15/RConn1
  13'3/LConn1 -- 16/RConn1

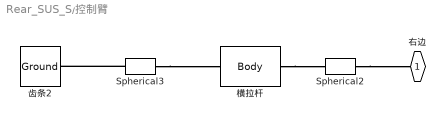
== system Rear_SUS_S/控制臂 ==
  Spherical2 : mblibv1/Joints/Spherical  LConnTagsString=__newl0  RConnTagsString=__newr0  UpdateFromCAD=off  NumSAPorts=0  CutJoint=off  MarkAsCut=off  Primitives=spherical  PrimitiveProps=S$WORLD$[0 0 0]$spherical  DialogClass=JointBlock  SAxis=[0 0 0]
  Spherical3 : mblibv1/Joints/Spherical  LConnTagsString=__newl0  RConnTagsString=__newr0  UpdateFromCAD=off  NumSAPorts=0  CutJoint=off  MarkAsCut=off  Primitives=spherical  PrimitiveProps=S$WORLD$[0 0 0]$spherical  DialogClass=JointBlock  SAxis=[0 0 0]
  横拉杆 : mblibv1/Bodies/Body  LConnTagsString=CS1  RConnTagsString=CS2  UpdateFromCAD=off  DialogClass=MechanicalBodyBlock  Mass=1  MassUnits=kg  InertiaUnits=kg*m^2  Inertia=eye(3)  Shape=Cylinder  ShapeDims=[1 1]  ShapeUnits=m  ShapeUse=false  Density=1  DensityUnits=kg/m^3  DensityUse=false  GraphicsMode=MACHINE_DEFAULT  BodyColorSelMode=MACHINE_DEFAULT  BodyColor=[1 0 0]  AttachedToCS=CG  CG=Left$CG$[(X11+X12)/2 (Y11+Y12)/2 (Z11+Z12)/2]$WORLD$WORLD$mm$[0 0 0]$Euler X-Y-Z$deg$WORLD$false$none  WorkingFrames=Left$CS1$[X11 Y11 Z11]$World$World$mm$[0 0 0]$Euler X-Y-Z$deg$WORLD$true$none#Right$CS2$[X12 Y12 Z12]$World$World$mm$[0 0 0]$Euler X-Y-Z$deg$WORLD$true$none  CGPos=[(X11+X12)/2 (Y11+Y12)/2 (Z11+Z12)/2]  CGRot=[0 0 0]  CS0Pos=[]  CS0Rot=[]  CS1Pos=[X11 Y11 Z11]  CS1Rot=[0 0 0]  CS2Pos=[X12 Y12 Z12]  CS2Rot=[0 0 0]  CS3Pos=[]  CS3Rot=[]  CS4Pos=[]  CS4Rot=[]  CS5Pos=[]  CS5Rot=[]  CS6Pos=[]  CS6Rot=[]  CS7Pos=[]  CS7Rot=[]  CS8Pos=[]  CS8Rot=[]  CS9Pos=[]  CS9Rot=[]  CS10Pos=[]  CS10Rot=[]  CS11Pos=[]  CS11Rot=[]  CS12Pos=[]  CS12Rot=[]  CS13Pos=[]  CS13Rot=[]  CS14Pos=[]  CS14Rot=[]  CS15Pos=[]  CS15Rot=[]  CS16Pos=[]  CS16Rot=[]  CS17Pos=[]  CS17Rot=[]  CS18Pos=[]  CS18Rot=[]  CS19Pos=[]  CS19Rot=[]  CS20Pos=[]  CS20Rot=[]
  齿条2 : mblibv1/Bodies/Ground  UpdateFromCAD=off  LeftPortType=env  RightPortType=workingframe  PhysicalDomain=Mechanical  DialogClass=GroundBlock  CoordPosition=[X11 Y11 Z11]  CoordPositionUnits=mm  StateVectorMgrId=-1  MachineId=[0 0]  ShowEnvPort=off  ParameterChecksum=[0 0 0 0]  TopologyChecksum=[0 0 0 0]
  右边 : PMIOPort  Port=1  Side=Right
  connections:
  横拉杆/RConn1 -- Spherical2/LConn1
  Spherical2/RConn1 -- 右边/RConn1
  Spherical3/LConn1 -- 齿条2/RConn1
  Spherical3/RConn1 -- 横拉杆/LConn1

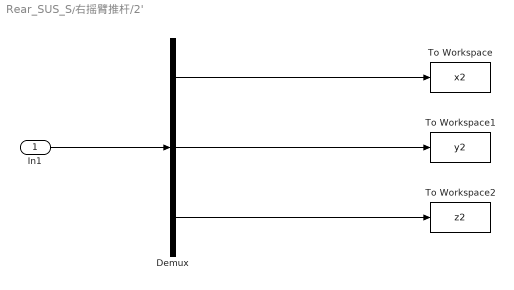
== system Rear_SUS_S/右摇臂推杆/2' ==
  In1 : Inport
  Demux : Demux  Outputs=3
  To Workspace : ToWorkspace  VariableName=x2  SampleTime=-1
  To Workspace1 : ToWorkspace  VariableName=y2  SampleTime=-1
  To Workspace2 : ToWorkspace  VariableName=z2  SampleTime=-1
  wires:
  In1/1 -> Demux/1
  Demux/3 -> To Workspace2/1
  Demux/1 -> To Workspace/1
  Demux/2 -> To Workspace1/1

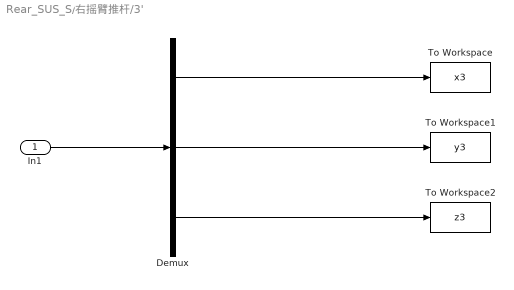
== system Rear_SUS_S/右摇臂推杆/3' ==
  In1 : Inport
  Demux : Demux  Outputs=3
  To Workspace : ToWorkspace  VariableName=x3  SampleTime=-1
  To Workspace1 : ToWorkspace  VariableName=y3  SampleTime=-1
  To Workspace2 : ToWorkspace  VariableName=z3  SampleTime=-1
  wires:
  Demux/2 -> To Workspace1/1
  Demux/1 -> To Workspace/1
  Demux/3 -> To Workspace2/1
  In1/1 -> Demux/1

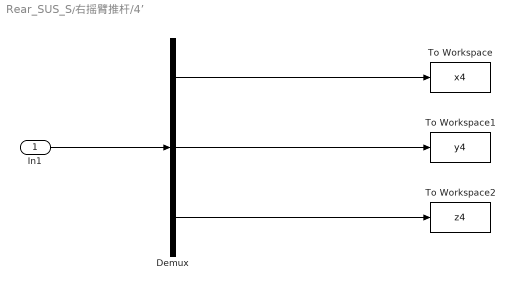
== system Rear_SUS_S/右摇臂推杆/4’ ==
  In1 : Inport
  Demux : Demux  Outputs=3
  To Workspace : ToWorkspace  VariableName=x4  SampleTime=-1
  To Workspace1 : ToWorkspace  VariableName=y4  SampleTime=-1
  To Workspace2 : ToWorkspace  VariableName=z4  SampleTime=-1
  wires:
  In1/1 -> Demux/1
  Demux/3 -> To Workspace2/1
  Demux/1 -> To Workspace/1
  Demux/2 -> To Workspace1/1

== system Rear_SUS_S/右摇臂推杆/5' ==
  In1 : Inport
  Demux : Demux  Outputs=3
  To Workspace : ToWorkspace  VariableName=x5  SampleTime=-1
  To Workspace1 : ToWorkspace  VariableName=y5  SampleTime=-1
  To Workspace2 : ToWorkspace  VariableName=z5  SampleTime=-1
  wires:
  Demux/2 -> To Workspace1/1
  Demux/1 -> To Workspace/1
  Demux/3 -> To Workspace2/1
  In1/1 -> Demux/1

== system Rear_SUS_S/右摇臂推杆/7' ==
  In1 : Inport
  Demux : Demux  Outputs=3
  To Workspace : ToWorkspace  VariableName=x7  SampleTime=-1
  To Workspace1 : ToWorkspace  VariableName=y7  SampleTime=-1
  To Workspace2 : ToWorkspace  VariableName=z7  SampleTime=-1
  wires:
  In1/1 -> Demux/1
  Demux/3 -> To Workspace2/1
  Demux/1 -> To Workspace/1
  Demux/2 -> To Workspace1/1

== system Rear_SUS_S/右测量/12坐标 ==
  In1 : Inport
  Demux : Demux  Outputs=3
  To Workspace : ToWorkspace  VariableName=X12  SampleTime=-1
  To Workspace1 : ToWorkspace  VariableName=Y12  SampleTime=-1
  To Workspace2 : ToWorkspace  VariableName=Z12  SampleTime=-1
  wires:
  Demux/2 -> To Workspace1/1
  Demux/1 -> To Workspace/1
  Demux/3 -> To Workspace2/1
  In1/1 -> Demux/1

== system Rear_SUS_S/右测量/14坐标1 ==
  In1 : Inport
  Demux : Demux  Outputs=3
  To Workspace : ToWorkspace  VariableName=X14  SampleTime=-1
  To Workspace1 : ToWorkspace  VariableName=Y14  SampleTime=-1
  To Workspace2 : ToWorkspace  VariableName=Z14  SampleTime=-1
  wires:
  In1/1 -> Demux/1
  Demux/3 -> To Workspace2/1
  Demux/1 -> To Workspace/1
  Demux/2 -> To Workspace1/1

== system Rear_SUS_S/右测量/15坐标2 ==
  In1 : Inport
  Demux : Demux  Outputs=3
  To Workspace : ToWorkspace  VariableName=X15  SampleTime=-1
  To Workspace1 : ToWorkspace  VariableName=Y15  SampleTime=-1
  To Workspace2 : ToWorkspace  VariableName=Z15  SampleTime=-1
  wires:
  Demux/2 -> To Workspace1/1
  Demux/1 -> To Workspace/1
  Demux/3 -> To Workspace2/1
  In1/1 -> Demux/1

== system Rear_SUS_S/右测量/16坐标1 ==
  In1 : Inport
  Demux : Demux  Outputs=3
  To Workspace : ToWorkspace  VariableName=X16  SampleTime=-1
  To Workspace1 : ToWorkspace  VariableName=Y16  SampleTime=-1
  To Workspace2 : ToWorkspace  VariableName=Z16  SampleTime=-1
  wires:
  In1/1 -> Demux/1
  Demux/3 -> To Workspace2/1
  Demux/1 -> To Workspace/1
  Demux/2 -> To Workspace1/1

== system Rear_SUS_S/右测量/2坐标 ==
  In1 : Inport
  Demux : Demux  Outputs=3
  To Workspace : ToWorkspace  VariableName=X2  SampleTime=-1
  To Workspace1 : ToWorkspace  VariableName=Y2  SampleTime=-1
  To Workspace2 : ToWorkspace  VariableName=Z2  SampleTime=-1
  wires:
  Demux/2 -> To Workspace1/1
  Demux/1 -> To Workspace/1
  Demux/3 -> To Workspace2/1
  In1/1 -> Demux/1

== system Rear_SUS_S/右测量/3坐标 ==
  In1 : Inport
  Demux : Demux  Outputs=3
  To Workspace : ToWorkspace  VariableName=X3  SampleTime=-1
  To Workspace1 : ToWorkspace  VariableName=Y3  SampleTime=-1
  To Workspace2 : ToWorkspace  VariableName=Z3  SampleTime=-1
  wires:
  In1/1 -> Demux/1
  Demux/3 -> To Workspace2/1
  Demux/1 -> To Workspace/1
  Demux/2 -> To Workspace1/1

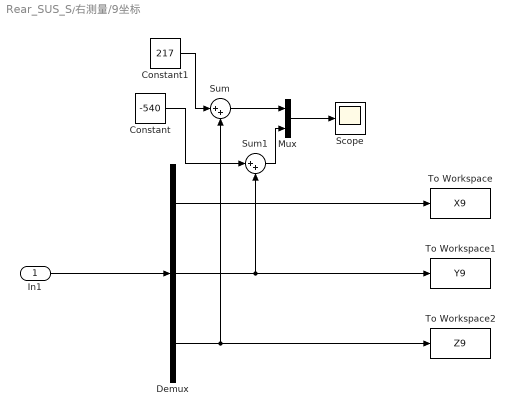
== system Rear_SUS_S/右测量/9坐标 ==
  In1 : Inport
  Constant : Constant  Value=-540
  Constant1 : Constant  Value=217
  Demux : Demux  Outputs=3
  Mux : Mux  Inputs=2
  Scope : Scope
      settings: TimeRange=10  YMin=-0.5  YMax=1
  Sum : Sum  Inputs=|++
  Sum1 : Sum  Inputs=|++
  To Workspace : ToWorkspace  VariableName=X9  SampleTime=-1
  To Workspace1 : ToWorkspace  VariableName=Y9  SampleTime=-1
  To Workspace2 : ToWorkspace  VariableName=Z9  SampleTime=-1
  wires:
  Demux/2 -> To Workspace1/1, Sum1/2
  Demux/1 -> To Workspace/1
  Demux/3 -> Sum/2, To Workspace2/1
  In1/1 -> Demux/1
  Mux/1 -> Scope/1
  Sum/1 -> Mux/1
  Sum1/1 -> Mux/2
  Constant1/1 -> Sum/1
  Constant/1 -> Sum1/1
